simulink subsystem "square_generator"  (R2019b)
settings: Solver=VariableStepAuto  StartTime=0.0  StopTime=10.0  RelTol=1e-3
libraries: quarc_library x1
settings Model: Creator=icpmoles  LastModifiedBy=icpmoles

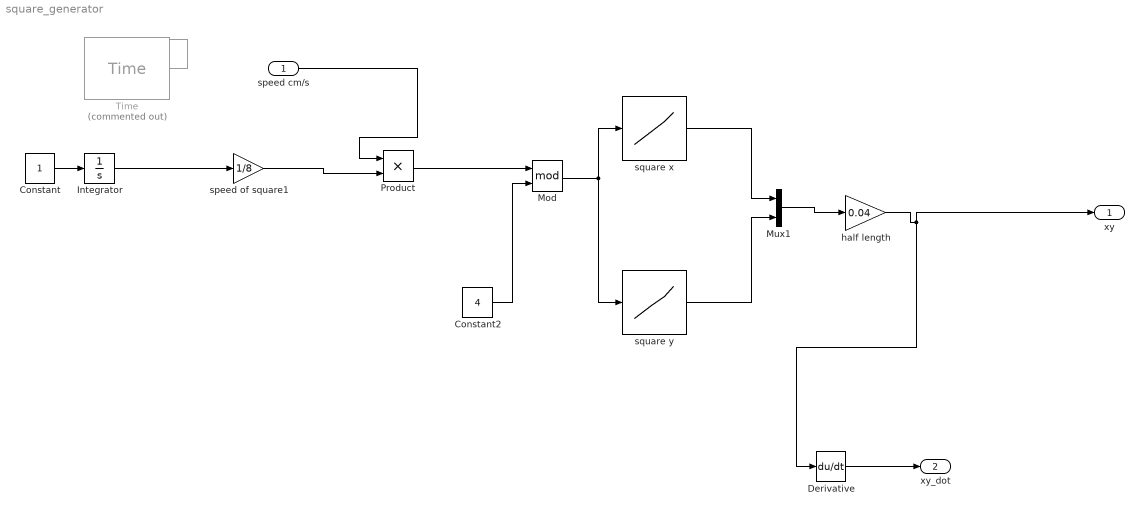
== system square_generator ==
  speed cm/s : Inport
  Constant : Constant
  Constant2 : Constant  Value=4
  Derivative : Derivative
  Integrator : Integrator
  Mod : Math  Operator=mod  SignedPower=off  SaturateOnIntegerOverflow=on
  Mux1 : Mux  Inputs=2
  Product : Product
  Time : quarc_library/Sources/Time/Time  Commented=on  time_source=Wall clock  sample_time=qc_get_step_size
  half length : Gain  Gain=0.04
  speed of square1 : Gain  Gain=1/8
  square x : Lookup_n-D  NumberOfTableDimensions=1  BreakpointsForDimension1=0:4  Table=[-1, 1 , 1 , -1 ,-1]  InternalRulePriority=Speed  RndMeth=Simplest  InputSameDT=on
  square y : Lookup_n-D  NumberOfTableDimensions=1  BreakpointsForDimension1=0:4  Table=[-1, -1 , 1 , 1 ,-1]  InternalRulePriority=Speed  RndMeth=Simplest  InputSameDT=on
  xy : Outport
  xy_dot : Outport  Port=2
  wires:
  speed of square1/1 -> Product/2
  half length/1 -> Derivative/1, xy/1
  square x/1 -> Mux1/1
  Mod/1 -> square y/1, square x/1
  Constant2/1 -> Mod/2
  Time/1 -> ?
  square y/1 -> Mux1/2
  Mux1/1 -> half length/1
  Derivative/1 -> xy_dot/1
  speed cm/s/1 -> Product/1
  Product/1 -> Mod/1
  Integrator/1 -> speed of square1/1
  Constant/1 -> Integrator/1
